simulink model "Gimbal_secondary_offsets"  (R2019b)
settings: Solver=ode5  StartTime=0.0  StopTime=inf  RelTol=1e-3
undefined symbols (not defined in the file): Serial_Port, Standard_Devices
libraries: custom_blocks x14, simulink x2, sldrtlib x2, simulink_extras x2
settings Model: Creator=guy-m  LastModifiedBy=guy-m
settings RTWCC: Description=Simulink Desktop Real-Time  SystemTargetFile=sldrt.tlc  TemplateMakefile=sldrt.tmf  RTWCompilerOptimization=on
settings CodeAppCC: MaxIdLength=95
settings SimulinkDesktopRealTimeCC: TargetPreCompLibLocation=C:\Program Files\MATLAB\R2019b\toolbox\sldrt\lib\win64  PreserveStateflowLocalDataDimensions=off

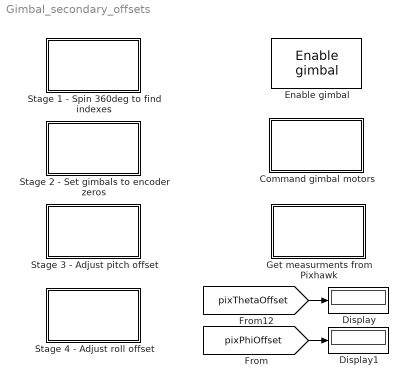
== system Gimbal_secondary_offsets ==
  Command gimbal motors : Subsystem
  Display : Display
  Display1 : Display
  Enable gimbal : custom_blocks/Enable gimbal
  Get measurments from Pixhawk : Subsystem
  Stage 1 - Spin 360deg to find indexes : Subsystem
  "Stage 2 - Set gimbals to encoder zeros " : Subsystem
  Stage 3 - Adjust pitch offset : Subsystem
  Stage 4 - Adjust roll offset : Subsystem
  wires:
  [pixThetaOffset] -> Display/1
  [pixPhiOffset] -> Display1/1

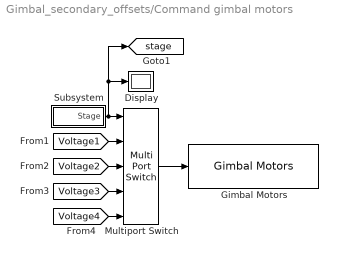
== system Gimbal_secondary_offsets/Command gimbal motors ==
  Display : Display
  Gimbal Motors : custom_blocks/Gimbal Motors
  Multiport Switch : MultiPortSwitch  DataPortOrder=Zero-based contiguous  Inputs=4  zeroidx=on
  Subsystem : Subsystem
  tag scope: stage=global
  wires:
  Subsystem/1(Stage) -> [stage], Display/1, Multiport Switch/1
  [Voltage4] -> Multiport Switch/5
  [Voltage2] -> Multiport Switch/3
  [Voltage1] -> Multiport Switch/2
  [Voltage3] -> Multiport Switch/4
  Multiport Switch/1 -> Gimbal Motors/1

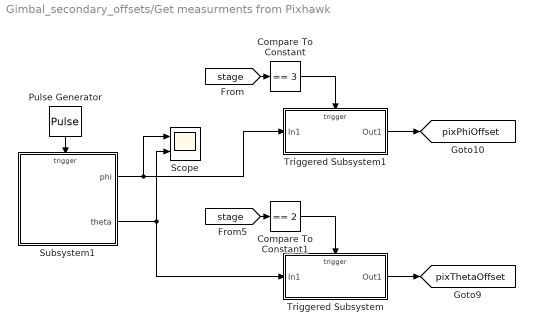
== system Gimbal_secondary_offsets/Get measurments from Pixhawk ==
  Compare To Constant : simulink/Logic and Bit Operations/Compare To Constant  relop===  const=3  OutDataTypeStr=boolean
  Compare To Constant1 : simulink/Logic and Bit Operations/Compare To Constant  relop===  const=2  OutDataTypeStr=boolean
  Pulse Generator : DiscretePulseGenerator  PulseType=Time based  Period=0.01  PulseWidth=50
  Scope : Scope  NumInputPorts=2
  Subsystem1 : Subsystem
  Triggered Subsystem : Subsystem  TreatAsAtomicUnit=on
  Triggered Subsystem1 : Subsystem  TreatAsAtomicUnit=on
  tag scope: pixPhiOffset=global, pixThetaOffset=global
  wires:
  Subsystem1/1(phi) -> Triggered Subsystem1/1(In1), Scope/1
  [stage] -> Compare To Constant1/1
  Triggered Subsystem/1(Out1) -> [pixThetaOffset]
  [stage] -> Compare To Constant/1
  Triggered Subsystem1/1(Out1) -> [pixPhiOffset]
  Pulse Generator/1 -> Subsystem1/Trigger
  Subsystem1/2(theta) -> Scope/2, Triggered Subsystem/1(In1)
  Compare To Constant1/1 -> Triggered Subsystem/Trigger
  Compare To Constant/1 -> Triggered Subsystem1/Trigger

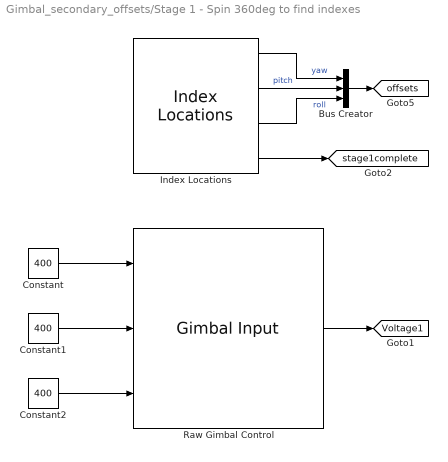
== system Gimbal_secondary_offsets/Stage 1 - Spin 360deg to find indexes ==
  Bus Creator : BusCreator  Inputs=3
  Constant : Constant  Value=400
  Constant1 : Constant  Value=400
  Constant2 : Constant  Value=400
  Index Locations : custom_blocks/Index Locations
  Raw Gimbal Control : custom_blocks/Gimbal Input  yawOffset=0  pitchOffset=0  rollOffset=0
  tag scope: Voltage1=global, offsets=global, stage1complete=global
  wires:
  Bus Creator/1 -> [offsets]
  Raw Gimbal Control/1 -> [Voltage1]
  Index Locations/4 -> [stage1complete]
  Constant1/1 -> Raw Gimbal Control/2
  Index Locations/1 -> Bus Creator/1  "yaw"
  Index Locations/3 -> Bus Creator/3  "roll"
  Constant2/1 -> Raw Gimbal Control/3
  Index Locations/2 -> Bus Creator/2  "pitch"
  Constant/1 -> Raw Gimbal Control/1

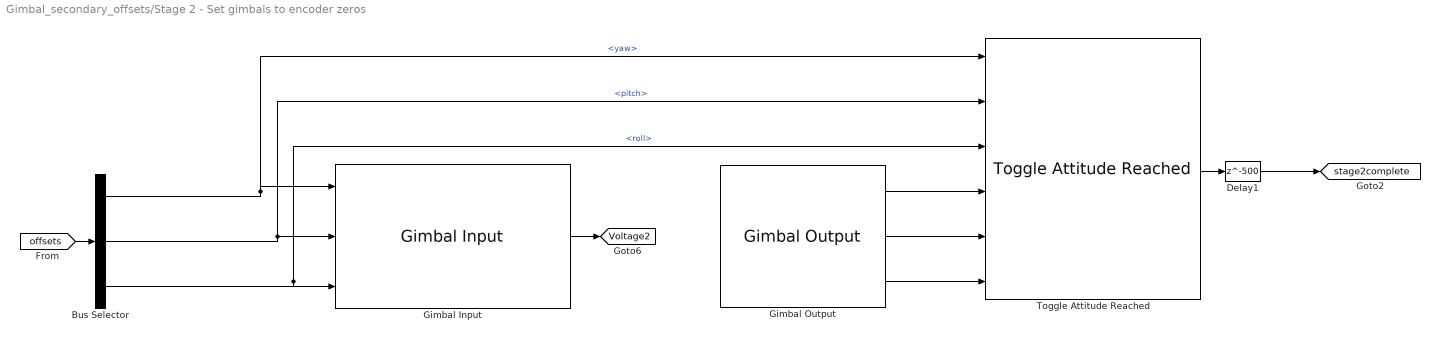
== system Gimbal_secondary_offsets/Stage 2 - Set gimbals to encoder zeros  ==
  Bus Selector : BusSelector  OutputSignals=yaw,pitch,roll
  Delay1 : Delay  DelayLength=500  InitialCondition=0  UseCircularBuffer=on
  Gimbal Input : custom_blocks/Gimbal Input  yawOffset=0  pitchOffset=0  rollOffset=0
  Gimbal Output : custom_blocks/Gimbal Output  yawOffset=0  pitchOffset=0  rollOffset=0
  Toggle Attitude Reached : custom_blocks/Toggle Attitude Reached
  tag scope: Voltage2=global, stage2complete=global
  wires:
  Delay1/1 -> [stage2complete]
  Toggle Attitude Reached/1 -> Delay1/1
  Gimbal Output/3 -> Toggle Attitude Reached/6
  Gimbal Output/2 -> Toggle Attitude Reached/5
  Gimbal Output/1 -> Toggle Attitude Reached/4
  Gimbal Input/1 -> [Voltage2]
  [offsets] -> Bus Selector/1
  Bus Selector/2 -> Gimbal Input/2, Toggle Attitude Reached/2  "<pitch>"
  Bus Selector/3 -> Gimbal Input/3, Toggle Attitude Reached/3  "<roll>"
  Bus Selector/1 -> Gimbal Input/1, Toggle Attitude Reached/1  "<yaw>"

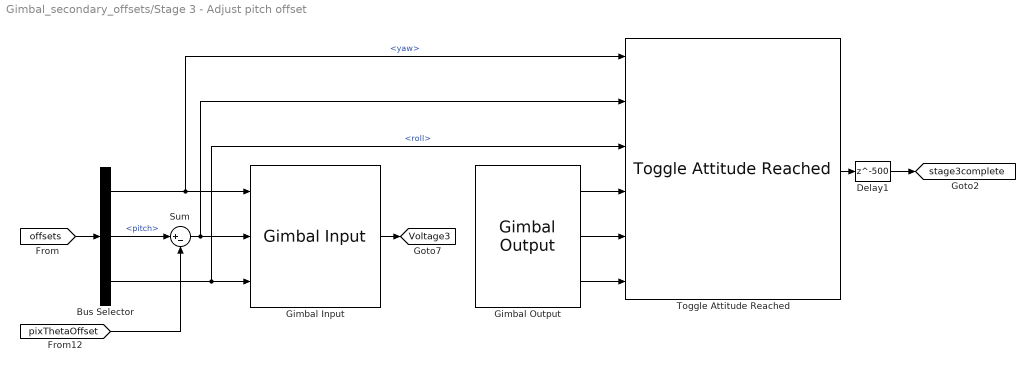
== system Gimbal_secondary_offsets/Stage 3 - Adjust pitch offset ==
  Bus Selector : BusSelector  OutputSignals=yaw,pitch,roll
  Delay1 : Delay  DelayLength=500  InitialCondition=0  UseCircularBuffer=on
  Gimbal Input : custom_blocks/Gimbal Input  yawOffset=0  pitchOffset=0  rollOffset=0
  Gimbal Output : custom_blocks/Gimbal Output  yawOffset=0  pitchOffset=0  rollOffset=0
  Sum : Sum  Inputs=|+-
  Toggle Attitude Reached : custom_blocks/Toggle Attitude Reached
  tag scope: Voltage3=global, stage3complete=global
  wires:
  Bus Selector/3 -> Gimbal Input/3, Toggle Attitude Reached/3  "<roll>"
  Bus Selector/1 -> Gimbal Input/1, Toggle Attitude Reached/1  "<yaw>"
  Toggle Attitude Reached/1 -> Delay1/1
  Gimbal Input/1 -> [Voltage3]
  Sum/1 -> Gimbal Input/2, Toggle Attitude Reached/2
  Bus Selector/2 -> Sum/1  "<pitch>"
  [pixThetaOffset] -> Sum/2
  [offsets] -> Bus Selector/1
  Delay1/1 -> [stage3complete]
  Gimbal Output/2 -> Toggle Attitude Reached/5
  Gimbal Output/3 -> Toggle Attitude Reached/6
  Gimbal Output/1 -> Toggle Attitude Reached/4

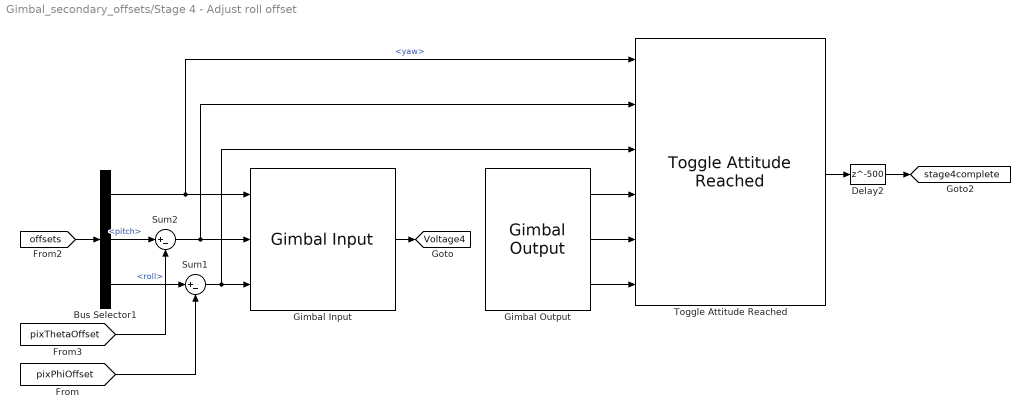
== system Gimbal_secondary_offsets/Stage 4 - Adjust roll offset ==
  Bus Selector1 : BusSelector  OutputSignals=yaw,pitch,roll
  Delay2 : Delay  DelayLength=500  InitialCondition=0  UseCircularBuffer=on
  Gimbal Input : custom_blocks/Gimbal Input  yawOffset=0  pitchOffset=0  rollOffset=0
  Gimbal Output : custom_blocks/Gimbal Output  yawOffset=0  pitchOffset=0  rollOffset=0
  Sum1 : Sum  Inputs=|+-
  Sum2 : Sum  Inputs=|+-
  Toggle Attitude Reached : custom_blocks/Toggle Attitude Reached
  tag scope: Voltage4=global, stage4complete=global
  wires:
  Gimbal Output/1 -> Toggle Attitude Reached/4
  [offsets] -> Bus Selector1/1
  Bus Selector1/2 -> Sum2/1  "<pitch>"
  Sum1/1 -> Gimbal Input/3, Toggle Attitude Reached/3
  Sum2/1 -> Gimbal Input/2, Toggle Attitude Reached/2
  [pixThetaOffset] -> Sum2/2
  Bus Selector1/1 -> Gimbal Input/1, Toggle Attitude Reached/1  "<yaw>"
  Delay2/1 -> [stage4complete]
  Gimbal Output/3 -> Toggle Attitude Reached/6
  Gimbal Output/2 -> Toggle Attitude Reached/5
  Toggle Attitude Reached/1 -> Delay2/1
  Gimbal Input/1 -> [Voltage4]
  [pixPhiOffset] -> Sum1/2
  Bus Selector1/3 -> Sum1/1  "<roll>"

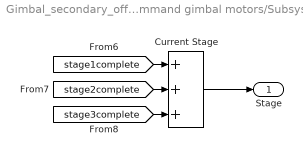
== system Gimbal_secondary_offsets/Command gimbal motors/Subsystem ==
  Current Stage : Sum  Inputs=3
  Stage : Outport
  wires:
  [stage2complete] -> Current Stage/2
  [stage3complete] -> Current Stage/3
  [stage1complete] -> Current Stage/1
  Current Stage/1 -> Stage/1

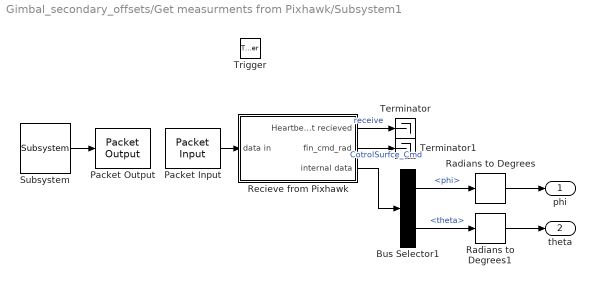
== system Gimbal_secondary_offsets/Get measurments from Pixhawk/Subsystem1 ==
  Trigger : TriggerPort  VariantControl=Variant  PortDimensions=1
  Bus Selector1 : BusSelector  OutputSignals=phi,theta
  Packet Input : sldrtlib/Packet Input  SampleTime=-1  MaxMissedTicks=10  ShowMissedTicks=off  YieldWhenWaiting=on  DrvName=Standard_Devices/Serial_Port  DrvAddress=3  DrvOptions=[115200 8 0 0 0 0 0 0]  PacketSize=17*4  DataTypes='17*single'  ShowReady=off  ShowError=off  PacketID=1  ByteOrder=1  ShowTimestamp=off
      settings: AttributesFormatString=Serial Port [3]  SourceProductName=Simulink Desktop Real-Time
  Packet Output : sldrtlib/Packet Output  SampleTime=-1  MaxMissedTicks=10  ShowMissedTicks=off  YieldWhenWaiting=on  DrvName=Standard_Devices/Serial_Port  DrvAddress=3  DrvOptions=[115200 8 0 0 0 0 0 0]  PacketSize=12*4  DataTypes='12*single'  ShowReady=off  ShowError=off  PacketID=1  ByteOrder=1  InitialValue=[]  FinalValue=[]
      settings: AttributesFormatString=Serial Port [3]  SourceProductName=Simulink Desktop Real-Time
  Radians to Degrees : simulink_extras/Transformations/Radians to Degrees
  Radians to Degrees1 : simulink_extras/Transformations/Radians to Degrees
  Recieve from Pixhawk : Subsystem
  Subsystem : custom_blocks/Subsystem
  Terminator : Terminator
  Terminator1 : Terminator
  phi : Outport
  theta : Outport  Port=2
  wires:
  Packet Input/1 -> Recieve from Pixhawk/1(data in)
  Subsystem/1 -> Packet Output/1
  Recieve from Pixhawk/3(internal data) -> Bus Selector1/1
  Recieve from Pixhawk/1(Heartbeat recieved) -> Terminator/1  "receive"
  Recieve from Pixhawk/2(fin_cmd_rad) -> Terminator1/1  "CotrolSurfce_Cmd"
  Bus Selector1/1 -> Radians to Degrees/1  "<phi>"
  Bus Selector1/2 -> Radians to Degrees1/1  "<theta>"
  Radians to Degrees/1 -> phi/1
  Radians to Degrees1/1 -> theta/1

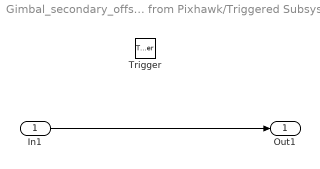
== system Gimbal_secondary_offsets/Get measurments from Pixhawk/Triggered Subsystem ==
  In1 : Inport
  Trigger : TriggerPort  VariantControl=Variant
  Out1 : Outport
  wires:
  In1/1 -> Out1/1

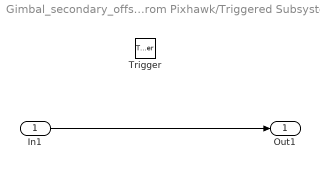
== system Gimbal_secondary_offsets/Get measurments from Pixhawk/Triggered Subsystem1 ==
  In1 : Inport
  Trigger : TriggerPort  VariantControl=Variant
  Out1 : Outport
  wires:
  In1/1 -> Out1/1

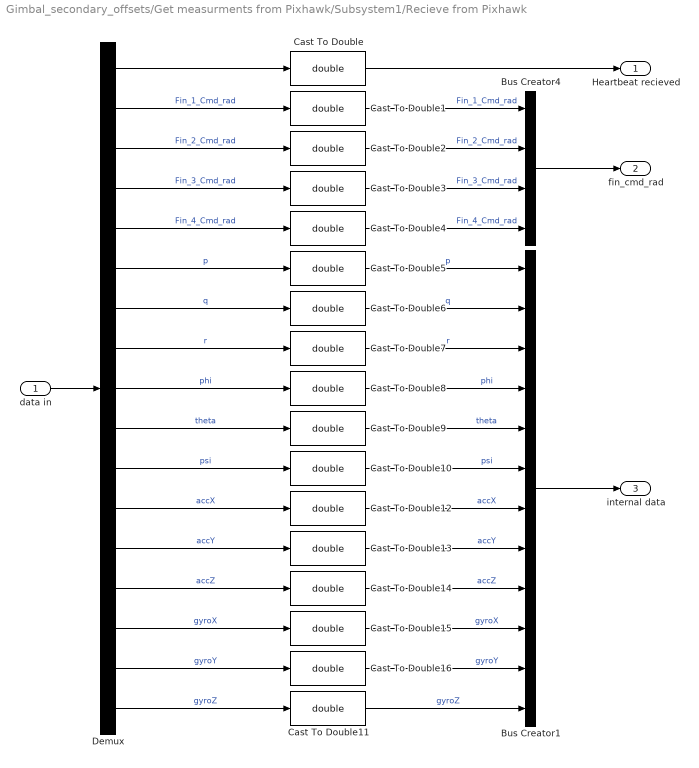
== system Gimbal_secondary_offsets/Get measurments from Pixhawk/Subsystem1/Recieve from Pixhawk ==
  data in : Inport
  Bus Creator1 : BusCreator  Inputs=12
  Bus Creator4 : BusCreator  Inputs=4  OutDataTypeStr=Bus: Control_Surface_Cmd_Bus
  Cast To Double{,1..16} (17 alike) : DataTypeConversion  OutDataTypeStr=double
  Demux : Demux  Outputs=17
  Heartbeat recieved : Outport
  fin_cmd_rad : Outport  Port=2
  internal data : Outport  Port=3
  wires:
  Cast To Double11/1 -> Bus Creator1/12  "gyroZ"
  Cast To Double16/1 -> Bus Creator1/11  "gyroY"
  Cast To Double15/1 -> Bus Creator1/10  "gyroX"
  Cast To Double14/1 -> Bus Creator1/9  "accZ"
  Cast To Double13/1 -> Bus Creator1/8  "accY"
  Cast To Double12/1 -> Bus Creator1/7  "accX"
  Demux/13 -> Cast To Double13/1  "accY"
  Demux/17 -> Cast To Double11/1  "gyroZ"
  Demux/16 -> Cast To Double16/1  "gyroY"
  Demux/15 -> Cast To Double15/1  "gyroX"
  Demux/14 -> Cast To Double14/1  "accZ"
  Demux/12 -> Cast To Double12/1  "accX"
  Cast To Double10/1 -> Bus Creator1/6  "psi"
  Cast To Double9/1 -> Bus Creator1/5  "theta"
  Cast To Double8/1 -> Bus Creator1/4  "phi"
  Cast To Double7/1 -> Bus Creator1/3  "r"
  Cast To Double6/1 -> Bus Creator1/2  "q"
  Cast To Double5/1 -> Bus Creator1/1  "p"
  Cast To Double4/1 -> Bus Creator4/4  "Fin_4_Cmd_rad"
  Cast To Double3/1 -> Bus Creator4/3  "Fin_3_Cmd_rad"
  Cast To Double2/1 -> Bus Creator4/2  "Fin_2_Cmd_rad"
  Cast To Double1/1 -> Bus Creator4/1  "Fin_1_Cmd_rad"
  Cast To Double/1 -> Heartbeat recieved/1
  Bus Creator1/1 -> internal data/1
  Bus Creator4/1 -> fin_cmd_rad/1
  Demux/6 -> Cast To Double5/1  "p"
  Demux/2 -> Cast To Double1/1  "Fin_1_Cmd_rad"
  Demux/3 -> Cast To Double2/1  "Fin_2_Cmd_rad"
  Demux/5 -> Cast To Double4/1  "Fin_4_Cmd_rad"
  Demux/4 -> Cast To Double3/1  "Fin_3_Cmd_rad"
  Demux/8 -> Cast To Double7/1  "r"
  Demux/9 -> Cast To Double8/1  "phi"
  Demux/10 -> Cast To Double9/1  "theta"
  Demux/11 -> Cast To Double10/1  "psi"
  Demux/7 -> Cast To Double6/1  "q"
  Demux/1 -> Cast To Double/1
  data in/1 -> Demux/1
